simulink model "aero_drag_test"  (R2016b)
settings: Solver=VariableStepAuto  StartTime=0.0  StopTime=10  RelTol=1e-3
undefined symbols (not defined in the file): fsw_params
libraries: GPS_time_lib x1, aero_drag_lib x1, time_coord_rotation_lib x1, tle2eci_coarse_lib x1
settings Model: Creator=Taylor  LastModifiedBy=bijan

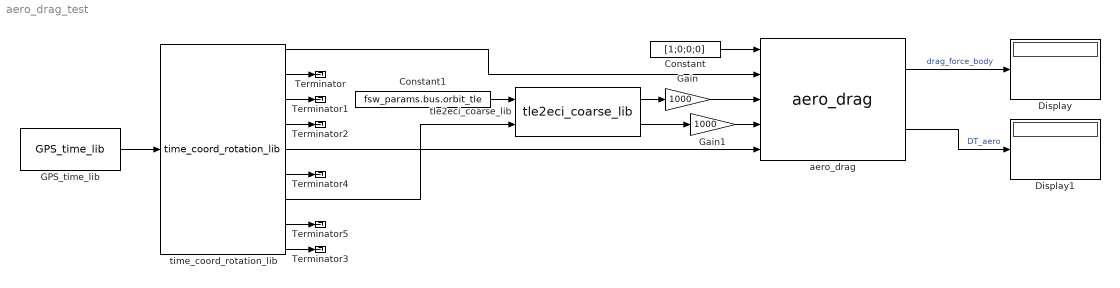
== system aero_drag_test ==
  Constant : Constant  Value=[1;0;0;0]
  Constant1 : Constant  Value=fsw_params.bus.orbit_tle
  Display : Display
  Display1 : Display
  GPS_time_lib : GPS_time_lib/GPS_time_lib
  Gain : Gain  Gain=1000
  Gain1 : Gain  Gain=1000
  Terminator{,1..5} (6 alike) : Terminator
  aero_drag : aero_drag_lib/aero_drag
  time_coord_rotation_lib : time_coord_rotation_lib/time_coord_rotation_lib
  tle2eci_coarse_lib : tle2eci_coarse_lib/tle2eci_coarse_lib
  wires:
  Constant/1 -> aero_drag/1
  time_coord_rotation_lib/5 -> aero_drag/5
  time_coord_rotation_lib/1 -> aero_drag/2
  GPS_time_lib/1 -> time_coord_rotation_lib/1
  time_coord_rotation_lib/2 -> Terminator/1
  time_coord_rotation_lib/3 -> Terminator1/1
  time_coord_rotation_lib/7 -> tle2eci_coarse_lib/2
  time_coord_rotation_lib/8 -> Terminator5/1
  Constant1/1 -> tle2eci_coarse_lib/1
  tle2eci_coarse_lib/2 -> Gain1/1
  tle2eci_coarse_lib/1 -> Gain/1
  aero_drag/1 -> Display/1  "drag_force_body"
  aero_drag/2 -> Display1/1  "DT_aero"
  Gain/1 -> aero_drag/3
  Gain1/1 -> aero_drag/4
  time_coord_rotation_lib/9 -> Terminator3/1
  time_coord_rotation_lib/4 -> Terminator2/1
  time_coord_rotation_lib/6 -> Terminator4/1
